simulink model "real_time_simulink_State_Space_Control"  (R2024b)
settings: Solver=ode5  StartTime=0.0  StopTime=5  FixedStep=0.001  RelTol=1e-3
InitFcn:
  | clear;
  | run("../Design12.m");
undefined symbols (not defined in the file): DiscIntNeverNeededParam, Estimator, K, National_Instruments, Nu, Nx, PCI, pulse2deg, t0, t1, V2deg
libraries: sldrtlib x3, simulink_extras x3, simulink x2
settings Model: SimulationMode=external  ExtModeTrigDuration=1000001  Creator=galeazzolu  LastModifiedBy=Banaan
settings DataIOCC: ReturnWorkspaceOutputs=off
settings HardwareCC: ProdBitPerLong=64  ProdHWDeviceType=Intel->x86-64 (Linux 64)
settings RTWCC: Description=Simulink Desktop Real-Time  SystemTargetFile=sldrt.tlc  TemplateMakefile=sldrt.tmf  RTWCompilerOptimization=on
settings CodeAppCC: MaxIdLength=95
settings SimulinkDesktopRealTimeCC: TargetLibSuffix=_sldrt.a  TargetPreCompLibLocation=C:\Program Files\MATLAB\R2024b\toolbox\sldrt\lib\win64  ParMdlRefBuildCompliant=on

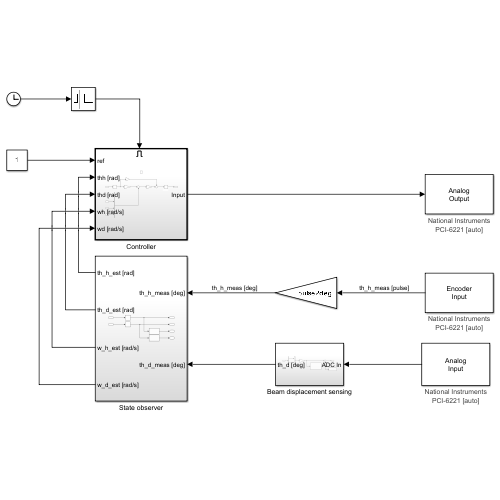
[thumbnail: Simulink's stored preview of the top-level diagram]
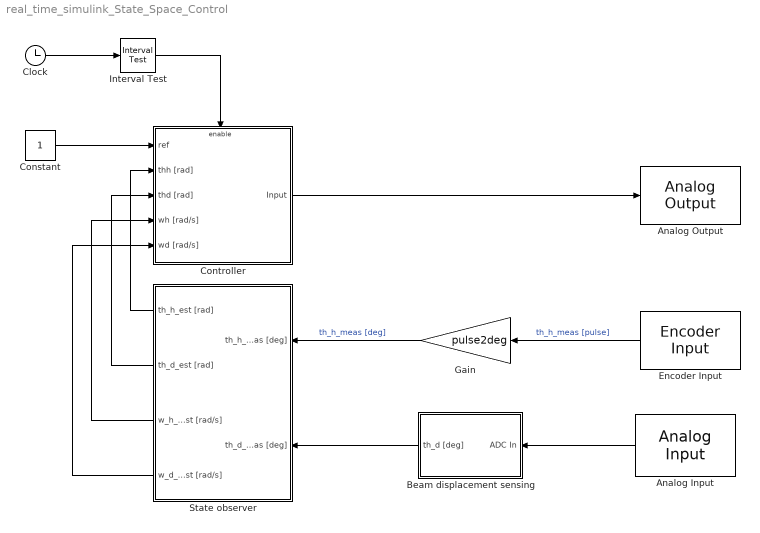
== system real_time_simulink_State_Space_Control ==
  Analog Input : sldrtlib/Analog Input  SampleTime=-1  MaxMissedTicks=10  ShowMissedTicks=off  YieldWhenWaiting=off  DrvName=National_Instruments/PCI-6221  DrvAddress=4294967295  DrvOptions=[0 0 0 2 0]  Channels=[1,2]  RangeMode=1  VoltRange=1  DataType=1
      settings: AttributesFormatString=National Instruments\nPCI-6221 [auto]
  Analog Output : sldrtlib/Analog Output  SampleTime=-1  MaxMissedTicks=10  ShowMissedTicks=off  YieldWhenWaiting=off  DrvName=National_Instruments/PCI-6221  DrvAddress=4294967295  DrvOptions=[0 0 0 2 0]  Channels=1  RangeMode=1  VoltRange=1  InitialValue=0  FinalValue=0
      settings: AttributesFormatString=National Instruments\nPCI-6221 [auto]
  Beam displacement sensing : Subsystem
  Clock : Clock
  Constant : Constant
  Controller : Subsystem
  Encoder Input : sldrtlib/Encoder Input  SampleTime=-1  MaxMissedTicks=10  ShowMissedTicks=off  YieldWhenWaiting=off  DrvName=National_Instruments/PCI-6221  DrvAddress=4294967295  DrvOptions=[0 0 0 2 0]  Channels=1  QuadMode=3  IndexPulse=1  InputFilter=Inf  DataType=1
      settings: AttributesFormatString=National Instruments\nPCI-6221 [auto]
  Gain : Gain  Gain=pulse2deg
  Interval Test : simulink/Logic and Bit Operations/Interval Test  IntervalClosedRight=on  uplimit=inf  IntervalClosedLeft=on  lowlimit=t1  OutDataTypeStr=boolean
  State observer : Subsystem
  wires:
  Beam displacement sensing/1(th_d [deg]) -> State observer/2(th_d_meas [deg])
  Gain/1 -> State observer/1(th_h_meas [deg])  "th_h_meas [deg]"
  State observer/2(th_d_est [rad]) -> Controller/3(thd [rad])
  State observer/1(th_h_est [rad]) -> Controller/2(thh [rad])
  Encoder Input/1 -> Gain/1  "th_h_meas [pulse]"
  State observer/4(w_d_est [rad/s]) -> Controller/5(wd [rad/s])
  Analog Input/1 -> Beam displacement sensing/1(ADC In)
  State observer/3(w_h_est [rad/s]) -> Controller/4(wh [rad/s])
  Clock/1 -> Interval Test/1
  Interval Test/1 -> Controller/Enable
  Constant/1 -> Controller/1(ref)
  Controller/1(Input) -> Analog Output/1

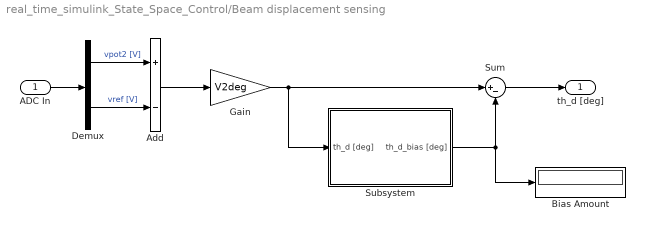
== system real_time_simulink_State_Space_Control/Beam displacement sensing ==
  ADC In : Inport
  Add : Sum  Inputs=+-
  Bias Amount : Display
  Demux : Demux  Outputs=2
  Gain : Gain  Gain=V2deg
  Subsystem : Subsystem
  Sum : Sum  Inputs=|+-
  th_d [deg] : Outport
  wires:
  ADC In/1 -> Demux/1
  Demux/1 -> Add/1  "vpot2 [V]"
  Demux/2 -> Add/2  "vref [V]"
  Add/1 -> Gain/1
  Gain/1 -> Subsystem/1(th_d [deg]), Sum/1
  Sum/1 -> th_d [deg]/1
  Subsystem/1(th_d_bias [deg]) -> Bias Amount/1, Sum/2

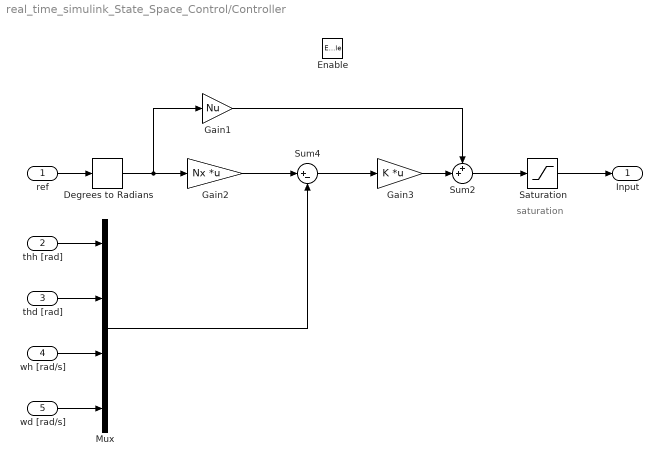
== system real_time_simulink_State_Space_Control/Controller ==
  note: saturation
  ref : Inport  PortDimensions=1
  thh [rad] : Inport  Port=2
  thd [rad] : Inport  Port=3
  wh [rad/s] : Inport  Port=4
  wd [rad/s] : Inport  Port=5
  Enable : EnablePort
  Degrees to Radians : simulink_extras/Transformations/Degrees to Radians
  Gain1 : Gain  Gain=Nu
  Gain2 : Gain  Gain=Nx  Multiplication=Matrix(K*u)
  Gain3 : Gain  Gain=K  Multiplication=Matrix(K*u)
  Mux : Mux
  Saturation : Saturate  UpperLimit=12  LowerLimit=-12  ZeroCross=off
  Sum2 : Sum  Inputs=++|
  Sum4 : Sum  Inputs=|+-
  Input : Outport  PortDimensions=1
  wires:
  thh [rad]/1 -> Mux/1
  thd [rad]/1 -> Mux/2
  Degrees to Radians/1 -> Gain1/1, Gain2/1
  Saturation/1 -> Input/1
  Sum2/1 -> Saturation/1
  Gain1/1 -> Sum2/1
  Gain3/1 -> Sum2/2
  Gain2/1 -> Sum4/1
  Mux/1 -> Sum4/2
  ref/1 -> Degrees to Radians/1
  Sum4/1 -> Gain3/1
  wd [rad/s]/1 -> Mux/4
  wh [rad/s]/1 -> Mux/3

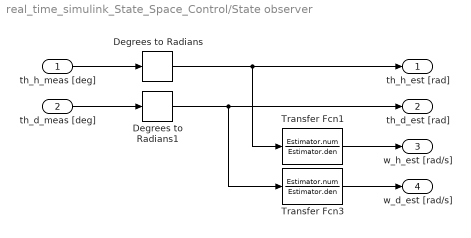
== system real_time_simulink_State_Space_Control/State observer ==
  th_h_meas [deg] : Inport
  th_d_meas [deg] : Inport  Port=2
  Degrees to Radians : simulink_extras/Transformations/Degrees to Radians
  Degrees to Radians1 : simulink_extras/Transformations/Degrees to Radians
  Transfer Fcn1 : TransferFcn  Numerator=Estimator.num  Denominator=Estimator.den
  Transfer Fcn3 : TransferFcn  Numerator=Estimator.num  Denominator=Estimator.den
  th_h_est [rad] : Outport
  th_d_est [rad] : Outport  Port=2
  w_h_est [rad/s] : Outport  Port=3
  w_d_est [rad/s] : Outport  Port=4
  wires:
  th_h_meas [deg]/1 -> Degrees to Radians/1
  Transfer Fcn1/1 -> w_h_est [rad/s]/1
  th_d_meas [deg]/1 -> Degrees to Radians1/1
  Transfer Fcn3/1 -> w_d_est [rad/s]/1
  Degrees to Radians/1 -> Transfer Fcn1/1, th_h_est [rad]/1
  Degrees to Radians1/1 -> Transfer Fcn3/1, th_d_est [rad]/1

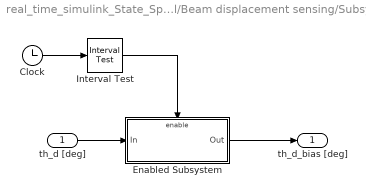
== system real_time_simulink_State_Space_Control/Beam displacement sensing/Subsystem ==
  th_d [deg] : Inport
  Clock : Clock
  Enabled Subsystem : Subsystem  TreatAsAtomicUnit=on
  Interval Test : simulink/Logic and Bit Operations/Interval Test  IntervalClosedRight=on  uplimit=t1  IntervalClosedLeft=on  lowlimit=t0  OutDataTypeStr=boolean
  th_d_bias [deg] : Outport
  wires:
  Interval Test/1 -> Enabled Subsystem/Enable
  Clock/1 -> Interval Test/1
  th_d [deg]/1 -> Enabled Subsystem/1(In)
  Enabled Subsystem/1(Out) -> th_d_bias [deg]/1

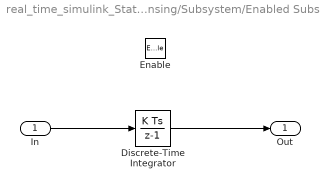
== system real_time_simulink_State_Space_Control/Beam displacement sensing/Subsystem/Enabled Subsystem ==
  In : Inport
  Enable : EnablePort
  Discrete-Time Integrator : DiscreteIntegrator  gainval=1/(t1-t0)  SampleTime=-1  ICPrevOutput=DiscIntNeverNeededParam  ICPrevScaledInput=DiscIntNeverNeededParam
  Out : Outport
  wires:
  In/1 -> Discrete-Time Integrator/1
  Discrete-Time Integrator/1 -> Out/1
